simulink model "testTXR"  (Simulink 7.9)
settings: Solver=ode45  StartTime=0.0  StopTime=10.0  RelTol=1e-3
libraries: commdigbbndpm3 x1, dspsrcs4 x1, commdigbbndam3 x1, commfilt2 x1, commtimrec2 x1
settings Model: Creator=ArunKB  LastModifiedBy=ArunKB

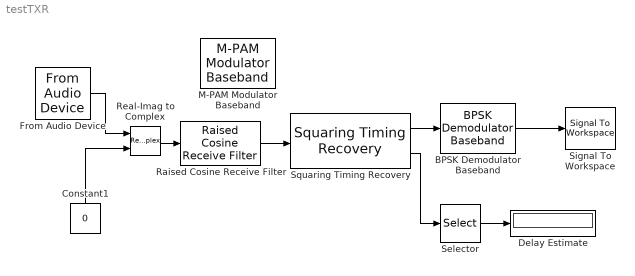
== system testTXR ==
  BPSK Demodulator Baseband : commdigbbndpm3/BPSK Demodulator Baseband  Ph=pi  DecType=Hard decision  VarSource=Dialog  Variance=1  outDtype=Inherit via internal rule  derotateFactorWordLen=16
  Constant1 : Constant  Value=0
  Delay Estimate : Display
  From Audio Device : dspsrcs4/From Audio Device  deviceName=Default  numChannels=1  sampleRate=8000  deviceDatatype=Determine from output data type  autoBufferSize=on  bufferSize=4096  queueDuration=1.0  frameSize=800  outputDatatype=double
  M-PAM Modulator Baseband : commdigbbndam3/M-PAM Modulator Baseband  M=4  InType=Integer  Enc=Gray  PowType=Min. distance between symbols  MinDist=2  AvgPow=1  PeakPow=1  outDtype=double  outWordLen=16  outUDDataType=sfix(16)  outFracLenMode=Best precision  outFracLen=15
  Raised Cosine Receive Filter : commfilt2/Raised Cosine Receive Filter  filtType=Square root  N=8  D=4  R=0.2  sampMode=Mute  saveAsFlag=0  rateMode=None  downFactor=8  downOffset=0  framing=Maintain input frame rate  InputProcessing=Columns as channels (frame based)  checkGain=Normalized  filterGain=1  checkCoeff=off  variableName=rcRxFilt  launchFVT=off  roundingMode=Floor  overflowMode=off
  Real-Imag to Complex : RealImagToComplex
  Selector : Selector  InputPortWidth=100  IndexOptions=Index vector (dialog)  Indices=1  OutputSizes=1
  Signal To Workspace : SignalToWorkspace  VariableName=yout
      settings: CopyFcn=dspblkcopystw(gcbh);
  Squaring Timing Recovery : commtimrec2/Squaring Timing Recovery  numSymb=100  sampPerSymb=8
  wires:
  From Audio Device/1 -> Real-Imag to Complex/1
  Constant1/1 -> Real-Imag to Complex/2
  Real-Imag to Complex/1 -> Raised Cosine Receive Filter/1
  Raised Cosine Receive Filter/1 -> Squaring Timing Recovery/1
  Squaring Timing Recovery/1 -> BPSK Demodulator Baseband/1
  Selector/1 -> Delay Estimate/1
  Squaring Timing Recovery/2 -> Selector/1
  BPSK Demodulator Baseband/1 -> Signal To Workspace/1
